simulink model "mavsim_chap3"  (R2018a)
settings: Solver=ode45  StartTime=0.0  StopTime=10000  RelTol=1e-3  EnableMultiTasking=on
InitFcn:
  | addpath('/Users/johnmcconnell/Desktop/mavsim_template_files-master/mavsim_simulink/chap2')
  | addpath('/Users/johnmcconnell/Desktop/mavsim_template_files-master/mavsim_simulink/parameters/')
  | aerosonde_parameters
  | addpath('/Users/johnmcconnell/Desktop/mavsim_template_files-master/mavsim_simulink/chap3')
  | addpath('/Users/johnmcconnell/Desktop/mavsim_template_files-master/mavsim_matlab/tools')
undefined symbols (not defined in the file or in its folder): drawSpacecraft
libraries: simulink x6
settings Model: Creator=beard  LastModifiedBy=johnmcconnell
settings DataIOCC: LimitDataPoints=on  SaveFormat=Array
settings OptimizationCC: ExpressionDepthLimit=2147483647  InitFltsAndDblsToZero=on  LifeSpan=inf
settings DebuggingCC: UnderspecifiedInitializationDetection=Classic  MergeDetectMultiDrivingBlocksExec=none  SolverPrmCheckMsg=warning  FcnCallInpInsideContextMsg=warning  AllowSymbolicDim=off  StateNameClashWarn=warning  SFUnexpectedBacktrackingDiag=warning  SFNoUnconditionalDefaultTransitionDiag=warning  SFExecutionAtInitializationDiag=none
settings HardwareCC: ProdBitPerPointer=32  ProdBitPerSizeT=32  ProdBitPerPtrDiffT=32  ProdLargestAtomicFloat=None  ProdIntDivRoundTo=Undefined  ProdEndianess=Unspecified  ProdWordSize=32  ProdHWDeviceType=32-bit Generic
settings ModelReferenceCC: PropagateSignalLabelsOutOfModel=off
settings CodeAppCC: StateflowObjectComments=on
settings GRTTargetCC: TargetLangStandard=C89/C90 (ANSI)  GeneratePreprocessorConditionals=Disable all  CombineOutputUpdateFcns=off  GRTInterface=on
settings ConfigComp: CovMetricSettings=dw  CovHtmlReporting=on  CovSaveCumulativeToWorkspaceVar=on  CovSaveSingleToWorkspaceVar=on  CovExternalEMLEnable=off  CovSFcnEnable=off

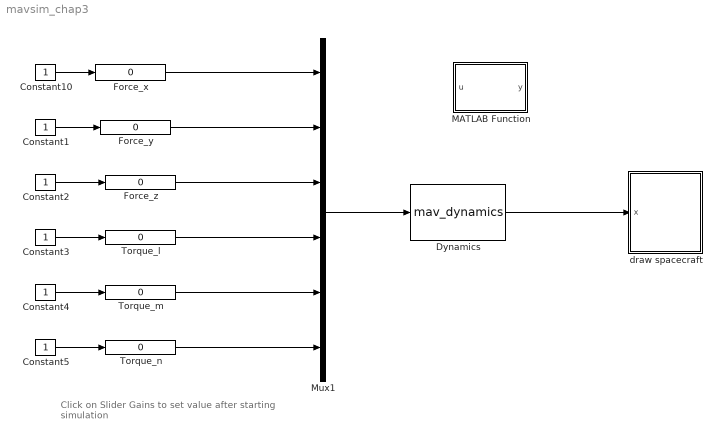
== system mavsim_chap3 ==
  note: Click on Slider Gains to set value
      | after starting simulation
  Constant{1..5,10} (6 alike) : Constant
  Dynamics : S-Function  FunctionName=mav_dynamics  Parameters=MAV  SFunctionDeploymentMode=off  EnableBusSupport=off
  Force_x : simulink/Math Operations/Slider Gain  gain=0  low=-1  high=1
  Force_y : simulink/Math Operations/Slider Gain  gain=0  low=-1  high=1
  Force_z : simulink/Math Operations/Slider Gain  gain=0  low=-1  high=1
  MATLAB Function : MATLAB Function  TreatAsAtomicUnit=on
  Mux1 : Mux  Inputs=6
  Torque_l : simulink/Math Operations/Slider Gain  gain=0  low=-0.1  high=0.1
  Torque_m : simulink/Math Operations/Slider Gain  gain=0  low=-0.1  high=0.1
  "Torque_n " : simulink/Math Operations/Slider Gain  gain=0  low=-0.1  high=0.1
  draw spacecraft : Subsystem
      mask init:
      | % Define the vertices (physical location of vertices
      |   V = [...
      | 	 1    1    0;... % point 1
      |      1   -1    0;... % point 2
      |     -1   -1    0;... % point 3
      |     -1    1    0;... % point 4
      | 	 1    1   -2;... % point 5
      |      1   -1   -2;... % point 6
      |     -1   -1   -2;... % point 7
      |     -1    1   -2;... % point 8
      | 	 1.5  1.5  0;... % point 9
      |      1.5 -1.5  0;... % point 10
      |     -1.5 -1.5  0;... % point 11
      |     -1.5  1.5  0;... % point 12
      |   ];
      | 
      | % define faces as a list of vertices numbered above
      |   F = [...
      |         1, 2,  6,  5;...  % front
      |         4, 3,  7,  8;...  % back
      |         1, 5,  8,  4;...  % right 
      |         2, 6,  7,  3;...  % left
      |         5, 6,  7,  8;...  % top
      |         9, 10, 11, 12;... % bottom
      |         ];
      | 
      | % define colors for each face    
      |   myred = [1, 0, 0];
      |   mygreen = [0, 1, 0];
      |   myblue = [0, 0, 1];
      |   myyellow = [1, 1, 0];
      |   mycyan = [0, 1, 1];
      | 
      |   patchcolors = [...
      |     myred;...    % front
      |     mygreen;...  % back
      |     myblue;...   % right
      |     myyellow;... % left
      |     mycyan;...   % top
      |     mycyan;...   % bottom
      |     ];
      mask Display: image(imread('tv.jpg'))
  wires:
  Constant5/1 -> "Torque_n "/1
  Constant10/1 -> Force_x/1
  Constant1/1 -> Force_y/1
  Constant2/1 -> Force_z/1
  Force_z/1 -> Mux1/3
  Force_y/1 -> Mux1/2
  Force_x/1 -> Mux1/1
  "Torque_n "/1 -> Mux1/6
  Constant4/1 -> Torque_m/1
  Torque_m/1 -> Mux1/5
  Constant3/1 -> Torque_l/1
  Torque_l/1 -> Mux1/4
  Mux1/1 -> Dynamics/1
  Dynamics/1 -> draw spacecraft/1(x)

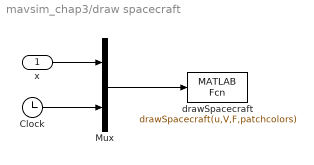
== system mavsim_chap3/draw spacecraft ==
  x : Inport
  Clock : Clock
  Mux : Mux  Inputs=2
  drawSpacecraft : MATLABFcn  MATLABFcn=drawSpacecraft(u,V,F,patchcolors)  OutputDimensions=0  SampleTime=0.1
  wires:
  Mux/1 -> drawSpacecraft/1
  x/1 -> Mux/1
  Clock/1 -> Mux/2

== matlab function mavsim_chap3/MATLAB Function ==
  data: u input; y output
function y = fcn(u)
classdef spacecraft_viewer < handle
%
%    Create spacecraft animation
%
%--------------------------------
properties
        body_handle
    	Vertices
    	Faces
    	facecolors
        plot_initialized
end
%--------------------------------
methods
%------constructor-----------
function self = spacecraft_viewer
            self.body_handle = [];
            [self.Vertices, self.Faces, self.facecolors] = self.define_spacecraft();
            self.plot_initialized = 0;           
end
%---------------------------
function self=update(self, state)
if self.plot_initialized==0
                figure(1); clf;
                self=self.drawBody(state.pn, state.pe, -state.h,...
                                   state.phi, state.theta, state.psi);
                title('Spacecraft')
                xlabel('East')
                ylabel('North')
                zlabel('-Down')
                view(32,47)  % set the vieew angle for figure
                axis([-10,10,-10,10,-10,10]);
hold on
grid on
                self.plot_initialized = 1;
else
                self=self.drawBody(state.pn, state.pe, -state.h,... 
                                   state.phi, state.theta, state.psi);
end
end
%---------------------------
function self = drawBody(self, pn, pe, pd, phi, theta, psi)
%Vertices = self.translate(self.Vertices, pn, pe, pd);
            Vertices = self.rotate(self.Vertices, phi, theta, psi);   % rotate rigid body  
            Vertices = self.translate(Vertices, pn, pe, pd);     % translate after rotation
% transform vertices from NED to ENU (for matlab rendering)
            R = [...
0, 1, 0;...
1, 0, 0;...
0, 0, -1;...
                ];
            Vertices = R*Vertices;
if isempty(self.body_handle)
                self.body_handle = patch('Vertices', Vertices', 'Faces', self.Faces,...
'FaceVertexCData',self.facecolors,...
'FaceColor','flat');
else
                set(self.body_handle,'Vertices',Vertices','Faces',self.Faces);
                drawnow
end
end 
%---------------------------
function pts=rotate(self, pts, phi, theta, psi)
% define rotation matrix (right handed)
            R_roll = [...
1, 0, 0;...
0, cos(phi), sin(phi);...
0, -sin(phi), cos(phi)];
            R_pitch = [...
                        cos(theta), 0, -sin(theta);...
0, 1, 0;...
                        sin(theta), 0, cos(theta)];
            R_yaw = [...
                        cos(psi), sin(psi), 0;...
                        -sin(psi), cos(psi), 0;...
0, 0, 1];
            R = R_roll*R_pitch*R_yaw;   % inertial to body
            R = R';  % body to inertial
% rotate vertices
            pts = R*pts;
end
%---------------------------
% translate vertices by pn, pe, pd
function pts = translate(self, pts, pn, pe, pd)
            pts = pts + repmat([pn;pe;pd],1,size(pts,2));
end
%---------------------------
function [V, F, colors] = define_spacecraft(self)
% Define the vertices (physical location of vertices)
            V = [...
%fusalage and nosecone
2    1    0;... % point 1
2   -1    0;... % point 2
2    1   -2;... % point 3
2   -1   -2;... % point 4
                -6   0   -1;... % point 5
3    0   -1;...%point 6
%wing
1   -3   -1;...%point 7
                -1   -3   -1;...%point 8
                -1    3   -1;...%point 9
1    3   -1;...%point 10
%tail wing
                -5   -1   -1;...%point 11
                -6   -1   -1;...%point 12
                -6    1    -1;...%point 13
                -5    1    -1;...%point 14
%tailfin
                -6   0  -1;...%point 15
                -5   0  -1;...%point 16
                -6   0  -3;...%point 17
            ]';
% define faces as a list of vertices numbered above
            F = [...
%fusalage
1, 2,  3,  4;...  % front
3, 4, 5, 3;...  % top
2, 4, 5, 2;...%left
1, 3, 5, 1;...%right
1, 2, 5, 1;...%bottom
%nosecone
3, 4, 6, 3;... %top
2, 4, 6, 2;...%left
1, 3, 6, 1;...%right
1, 2, 6, 1;...%bottom
%wing
7, 8, 9, 10;...
%tailwing
11, 12, 13, 14;...
%tailfin
15, 16, 17, 15;...
                    ];
% define colors for each face    
            myred = [1, 0, 0];
            mygreen = [0, 1, 0];
            myblue = [0, 0, 1];
            myyellow = [1, 1, 0];
            mycyan = [0, 1, 1];
            colors = [...
%fusalage
                myyellow;... % front
                myblue;...   % back
                myblue;...   % right
                myblue;...   % left
                myblue;...   % top
%nosecone
                myblue;... %top
                myblue;...
                myblue;...
                myblue;...
%wing
                mygreen;...  
%tailwing
                myyellow;...
%tailfin
                myred;...
                ];
end
end
end
